simulink model "WalshCodeCacher"  (R2024b)
settings: Solver=VariableStepAuto  StartTime=0.0  StopTime=1  RelTol=1e-3
StopFcn:
  | myDictionaryObj = Simulink.data.dictionary.open('ConfigData.sldd');
  | dDataSectObj = getSection(myDictionaryObj,'Design Data');
  | cacheObj = getEntry(dDataSectObj,'WalshCodeCache');
  | setValue(cacheObj,out.WalshCodeCache.Data);
model workspace (MAT data in the model file):
  WalshCodeCache_Draft = 0
values from neighbouring files (symbols this model uses):
  CanaryDataRate = 100.0    [ConfigData.sldd]
  PreConvolveDownsample = 32.0    [ConfigData.sldd]
  SampleRate = 48000.0    [ConfigData.sldd]
  WalshCodeIndex = 3.0 9.0    [ConfigData.sldd]
libraries: dspsigops x2, commseqgen3 x2
settings Model: DataDictionary=ConfigData.sldd  Creator=calum  LastModifiedBy=calum

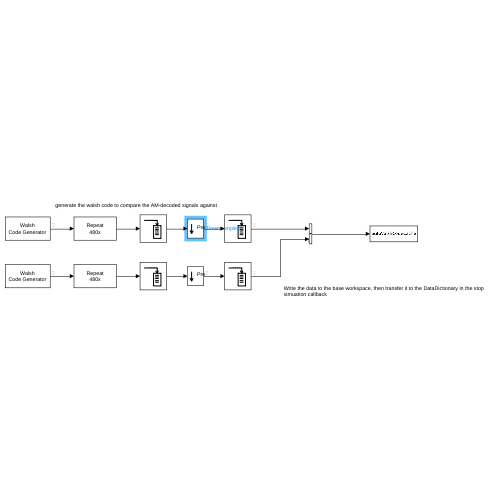
[thumbnail: Simulink's stored preview of the top-level diagram]
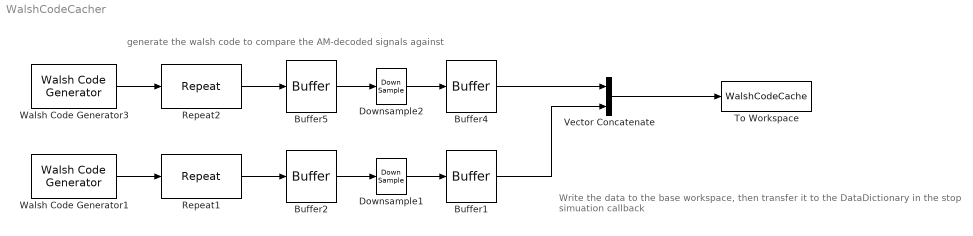
== system WalshCodeCacher ==
  note: generate the walsh code to compare the AM-decoded signals against
  note: Write the data to the base workspace, then transfer it to the DataDictionary in the stop simuation callback
  Buffer1 : Buffer  N=ceil(SampleRate/32/CanaryDataRate*16)  OutputFrames=off
  Buffer2 : Buffer  N=32  OutputFrames=off
  Buffer4 : Buffer  N=ceil(SampleRate/32/CanaryDataRate*16)  OutputFrames=off
  Buffer5 : Buffer  N=32  OutputFrames=off
  Downsample1 : DownSample  N=PreConvolveDownsample
  Downsample2 : DownSample  N=PreConvolveDownsample
  Repeat1 : dspsigops/Repeat  FactorSource=Dialog parameter  N=SampleRate/CanaryDataRate  Nmax=16  InputProcessing=Columns as channels (frame based)  RateOptions=Allow multirate processing  ic=0  mode=Unused parameter value
      settings: LibrarySourceBlock=commsequence2/Repeat
  Repeat2 : dspsigops/Repeat  FactorSource=Dialog parameter  N=SampleRate/CanaryDataRate  Nmax=16  InputProcessing=Columns as channels (frame based)  RateOptions=Allow multirate processing  ic=0  mode=Unused parameter value
      settings: LibrarySourceBlock=commsequence2/Repeat
  To Workspace : ToWorkspace  VariableName=WalshCodeCache  SaveFormat=Timeseries  SampleTime=-1
      settings: MaxDataPoints=1
  Vector Concatenate : Concatenate  Mode=Multidimensional array  ConcatenateDimension=2
  Walsh Code Generator1 : commseqgen3/Walsh Code Generator  Length=16  Index=WalshCodeIndex(2)  SampleTime=1/CanaryDataRate  SamplesPerFrame=1  OutputDataType=double  SimulateUsing=Code generation
  Walsh Code Generator3 : commseqgen3/Walsh Code Generator  Length=16  Index=WalshCodeIndex(1)  SampleTime=1/CanaryDataRate  SamplesPerFrame=1  OutputDataType=double  SimulateUsing=Code generation
  wires:
  Buffer5/1 -> Downsample2/1
  Repeat2/1 -> Buffer5/1
  Downsample2/1 -> Buffer4/1
  Walsh Code Generator3/1 -> Repeat2/1
  Buffer2/1 -> Downsample1/1
  Repeat1/1 -> Buffer2/1
  Downsample1/1 -> Buffer1/1
  Walsh Code Generator1/1 -> Repeat1/1
  Buffer4/1 -> Vector Concatenate/1
  Buffer1/1 -> Vector Concatenate/2
  Vector Concatenate/1 -> To Workspace/1
